simulink model "ProblemNo_4"  (R2020b)
settings: Solver=VariableStepAuto  StartTime=0.0  StopTime=10.0  RelTol=1e-3
settings Model: Creator=Pavan  LastModifiedBy=Pavan

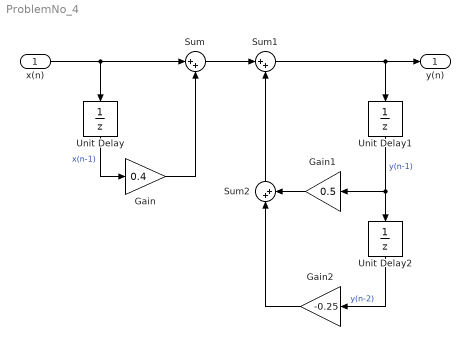
== system ProblemNo_4 ==
  x(n) : Inport
  Gain : Gain  Gain=0.4
  Gain1 : Gain  Gain=0.5
  Gain2 : Gain  Gain=-0.25
  Sum : Sum  Inputs=|++
  Sum1 : Sum  Inputs=|++
  Sum2 : Sum  Inputs=|++
  Unit Delay : UnitDelay  SampleTime=-1  HasFrameUpgradeWarning=on
  Unit Delay1 : UnitDelay  SampleTime=-1  HasFrameUpgradeWarning=on
  Unit Delay2 : UnitDelay  SampleTime=-1  HasFrameUpgradeWarning=on
  y(n) : Outport
  wires:
  x(n)/1 -> Sum/1, Unit Delay/1
  Unit Delay/1 -> Gain/1  "x(n-1)"
  Gain/1 -> Sum/2
  Sum/1 -> Sum1/1
  Sum1/1 -> y(n)/1, Unit Delay1/1
  Unit Delay1/1 -> Unit Delay2/1, Gain1/1  "y(n-1)"
  Sum2/1 -> Sum1/2
  Gain1/1 -> Sum2/2
  Gain2/1 -> Sum2/1
  Unit Delay2/1 -> Gain2/1  "y(n-2)"
